simulink model "Q5_withfault_observer"  (R2021b)
settings: Solver=ode45  StartTime=0.0  StopTime=5  MaxStep=2e-3  MinStep=1e-3  RelTol=1e-4  EnableMultiTasking=on
settings Model: Creator=samim  LastModifiedBy=user
settings SolverCC: AlgebraicLoopSolver=TrustRegion
settings DataIOCC: LimitDataPoints=on  SaveFormat=Array  ReturnWorkspaceOutputs=off
settings OptimizationCC: ExpressionDepthLimit=2147483647  LifeSpan=inf
settings DebuggingCC: UnderspecifiedInitializationDetection=Classic  MergeDetectMultiDrivingBlocksExec=none  SolverPrmCheckMsg=warning  StateNameClashWarn=warning  SFUnexpectedBacktrackingDiag=warning  SFNoUnconditionalDefaultTransitionDiag=warning  SFExecutionAtInitializationDiag=none  SFMachineParentedDataDiag=warning  ArithmeticOperatorsInVariantConditions=warning
settings HardwareCC: ProdBitPerPointer=32  ProdBitPerSizeT=32  ProdBitPerPtrDiffT=32  ProdLargestAtomicFloat=None  ProdIntDivRoundTo=Undefined  ProdEndianess=Unspecified  ProdWordSize=32  ProdHWDeviceType=32-bit Generic
settings ModelReferenceCC: PropagateSignalLabelsOutOfModel=off
settings SFSimCC: SimUseLocalCustomCode=off  CustomCodeUndefinedFunction=UseInterfaceOnly
settings RTWCC: RTWUseLocalCustomCode=off
settings CodeAppCC: StateflowObjectComments=on
settings GRTTargetCC: TargetLangStandard=C89/C90 (ANSI)
settings ConfigComp: CovMetricSettings=dw  CovSaveCumulativeToWorkspaceVar=on  CovSaveSingleToWorkspaceVar=on  CovExternalEMLEnable=off

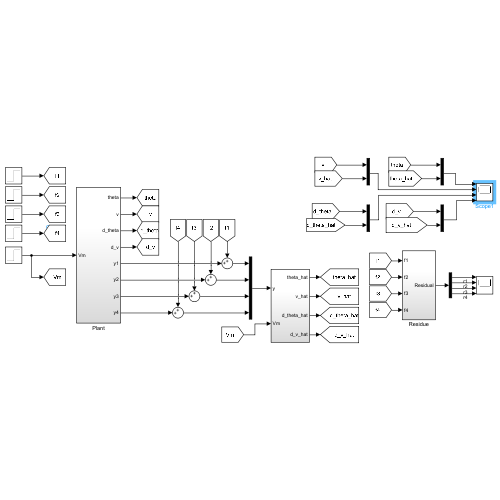
[thumbnail: Simulink's stored preview of the top-level diagram]
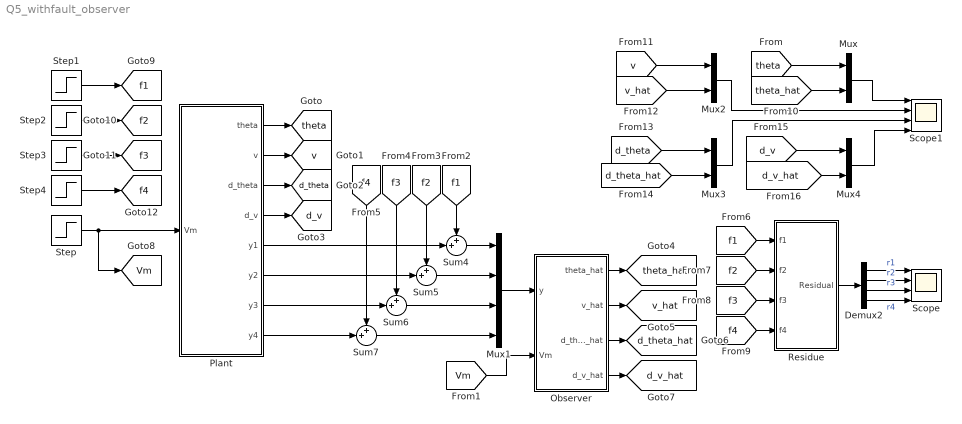
== system Q5_withfault_observer ==
  Demux2 : Demux
  Mux{,2..4} (4 alike) : Mux  Inputs=2
  Mux1 : Mux
  Observer : Subsystem
  Plant : Subsystem
  Residue : Subsystem
  Scope : Scope  NumInputPorts=4
  Scope1 : Scope  NumInputPorts=4
  Step{,1..3} (4 alike) : Step  Time=0  After=0  SampleTime=0
  Step4 : Step  Time=2  After=2  SampleTime=0
  Sum{4..7} (4 alike) : Sum  Inputs=++|
  tag scope: Vm=global, d_theta=global, d_theta_hat=global, d_v=global, d_v_hat=global, f1=global, f2=global, f3=global, f4=global, theta=global, theta_hat=global, v=global, v_hat=global
  wires:
  Demux2/1 -> Scope/1  "r1"
  Demux2/2 -> Scope/2  "r2"
  Demux2/3 -> Scope/3  "r3"
  Demux2/4 -> Scope/4  "r4"
  Step/1 -> [Vm], Plant/1(Vm)
  Mux1/1 -> Observer/1(y)
  Plant/8(y4) -> Sum7/2
  Plant/7(y3) -> Sum6/2
  Plant/6(y2) -> Sum5/2
  Plant/5(y1) -> Sum4/2
  Sum4/1 -> Mux1/1
  Sum5/1 -> Mux1/2
  Sum6/1 -> Mux1/3
  Sum7/1 -> Mux1/4
  Plant/1(theta) -> [theta]
  Plant/2(v) -> [v]
  Plant/4(d_v) -> [d_v]
  Plant/3(d_theta) -> [d_theta]
  Observer/1(theta_hat) -> [theta_hat]
  Observer/2(v_hat) -> [v_hat]
  Observer/3(d_theta_hat) -> [d_theta_hat]
  Observer/4(d_v_hat) -> [d_v_hat]
  Step1/1 -> [f1]
  Step2/1 -> [f2]
  Step3/1 -> [f3]
  Step4/1 -> [f4]
  [f4] -> Sum7/1
  [f3] -> Sum6/1
  [f2] -> Sum5/1
  [f1] -> Sum4/1
  Residue/1(Residual) -> Demux2/1
  [f1] -> Residue/1(f1)
  [f2] -> Residue/2(f2)
  [f3] -> Residue/3(f3)
  [f4] -> Residue/4(f4)
  [theta_hat] -> Mux/2
  [theta] -> Mux/1
  [Vm] -> Observer/2(Vm)
  [v_hat] -> Mux2/2
  [v] -> Mux2/1
  [d_theta_hat] -> Mux3/2
  [d_theta] -> Mux3/1
  [d_v_hat] -> Mux4/2
  [d_v] -> Mux4/1
  Mux/1 -> Scope1/1
  Mux3/1 -> Scope1/3
  Mux2/1 -> Scope1/2
  Mux4/1 -> Scope1/4

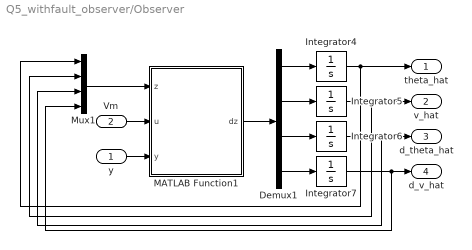
== system Q5_withfault_observer/Observer ==
  y : Inport
  Vm : Inport  Port=2
  Demux1 : Demux
  Integrator{4..7} (4 alike) : Integrator
  MATLAB Function1 : MATLAB Function  TreatAsAtomicUnit=on
  Mux1 : Mux
  theta_hat : Outport
  v_hat : Outport  Port=2
  d_theta_hat : Outport  Port=3
  d_v_hat : Outport  Port=4
  wires:
  MATLAB Function1/1(dz) -> Demux1/1
  Mux1/1 -> MATLAB Function1/1(z)
  Demux1/1 -> Integrator4/1
  Demux1/2 -> Integrator5/1
  Demux1/3 -> Integrator6/1
  Demux1/4 -> Integrator7/1
  Integrator5/1 -> Mux1/2, v_hat/1
  Integrator6/1 -> Mux1/3, d_theta_hat/1
  Integrator7/1 -> Mux1/4, d_v_hat/1
  y/1 -> MATLAB Function1/3(y)
  Integrator4/1 -> Mux1/1, theta_hat/1
  Vm/1 -> MATLAB Function1/2(u)

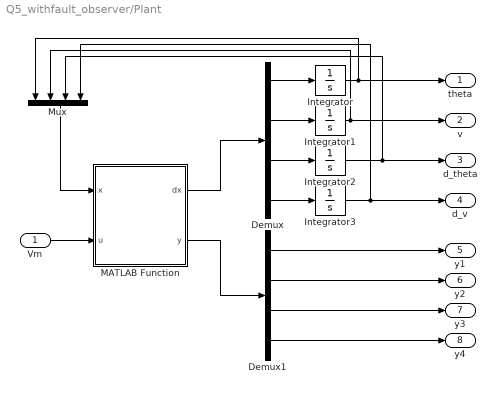
== system Q5_withfault_observer/Plant ==
  Vm : Inport
  Demux : Demux
  Demux1 : Demux
  Integrator{,1..3} (4 alike) : Integrator
  MATLAB Function : MATLAB Function  TreatAsAtomicUnit=on
  Mux : Mux
  theta : Outport
  v : Outport  Port=2
  d_theta : Outport  Port=3
  d_v : Outport  Port=4
  y1 : Outport  Port=5
  y2 : Outport  Port=6
  y3 : Outport  Port=7
  y4 : Outport  Port=8
  wires:
  Vm/1 -> MATLAB Function/2(u)
  Mux/1 -> MATLAB Function/1(x)
  Demux/1 -> Integrator/1
  Demux/2 -> Integrator1/1
  Demux/3 -> Integrator2/1
  Demux/4 -> Integrator3/1
  Integrator/1 -> theta/1, Mux/1
  Integrator1/1 -> v/1, Mux/2
  Integrator2/1 -> d_theta/1, Mux/3
  Integrator3/1 -> d_v/1, Mux/4
  MATLAB Function/1(dx) -> Demux/1
  Demux1/1 -> y1/1
  Demux1/2 -> y2/1
  Demux1/3 -> y3/1
  Demux1/4 -> y4/1
  MATLAB Function/2(y) -> Demux1/1

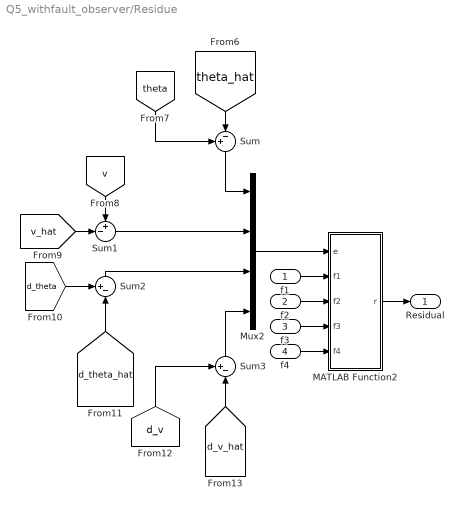
== system Q5_withfault_observer/Residue ==
  f1 : Inport
  f2 : Inport  Port=2
  f3 : Inport  Port=3
  f4 : Inport  Port=4
  MATLAB Function2 : MATLAB Function  TreatAsAtomicUnit=on
  Mux2 : Mux
  Sum{,1..3} (4 alike) : Sum  Inputs=+-|
  Residual : Outport
  wires:
  MATLAB Function2/1(r) -> Residual/1
  Sum/1 -> Mux2/1
  Mux2/1 -> MATLAB Function2/1(e)
  [theta_hat] -> Sum/2
  [theta] -> Sum/1
  [v] -> Sum1/1
  [v_hat] -> Sum1/2
  [d_v] -> Sum3/1
  Sum1/1 -> Mux2/2
  Sum3/1 -> Mux2/4
  [d_v_hat] -> Sum3/2
  [d_theta_hat] -> Sum2/2
  Sum2/1 -> Mux2/3
  [d_theta] -> Sum2/1
  f2/1 -> MATLAB Function2/3(f2)
  f3/1 -> MATLAB Function2/4(f3)
  f1/1 -> MATLAB Function2/2(f1)
  f4/1 -> MATLAB Function2/5(f4)

== matlab function Q5_withfault_observer/Observer/MATLAB Function1 ==
  data: z input; u input; y input; dz output
function dz = observer(z,u,y)
dz = zeros(4,1);
A = [0 0 1 0;0 0 0 1;0 483.1312 -28.2625 0;0 -837.2130 28.2625 0];
B = [0;0;49.7076;-49.7076];
C = eye(4);
L_p = [5 -1 1 0;1 5 0 1;0 483.1312 -20.2625 -0.5;0 -837.213 28.7625 8];
temp = (A-L_p*C)*z;
temp2 = B*u;
temp3 = L_p*y;
dz = temp(:,1)+temp2(:,1)+temp3(:,1);
end

== matlab function Q5_withfault_observer/Plant/MATLAB Function ==
  data: dx output; y output; x input; u input
function [dx, y] = plant(x,u)
dx = zeros(4,1);
A = [0 0 1 0;0 0 0 1;0 483.1312 -28.2625 0;0 -837.2130 28.2625 0];
B = [0;0;49.7076;-49.7076];
C = eye(4);
temp = A*x;
temp2 = B*u;
dx = temp(:,1) + temp2(:,1);
y = C*x;
%y = size(dx,1);
end

== matlab function Q5_withfault_observer/Residue/MATLAB Function2 ==
  data: e input; f1 input; r output; f2 input; f3 input; f4 input
function r  = residue(e,f1,f2,f3,f4)
L1 = eye(4); L2 = -L1; Df = eye(4);
f = [f1;f2;f3;f4];
temp2 = L1*e;
temp3 = L2*Df*f;
r = temp2(:,1) + temp3(:,1);
end
